simulink model "evse_full_shit"  (R2023b)
settings: Solver=VariableStepAuto  StartTime=0.0  StopTime=5  RelTol=1e-3
settings Model: Creator=dawid  LastModifiedBy=dawid
settings OptimizationCC: BooleanDataType=off

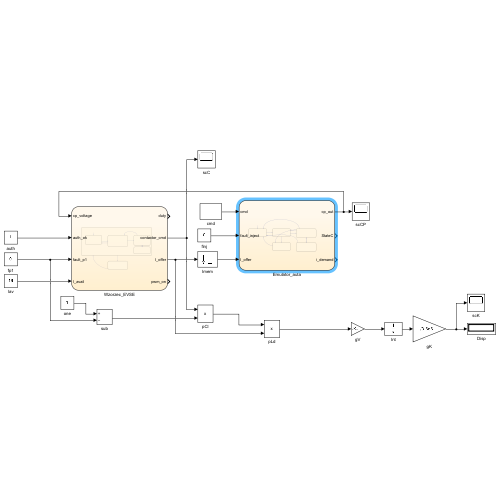
[thumbnail: Simulink's stored preview of the top-level diagram]
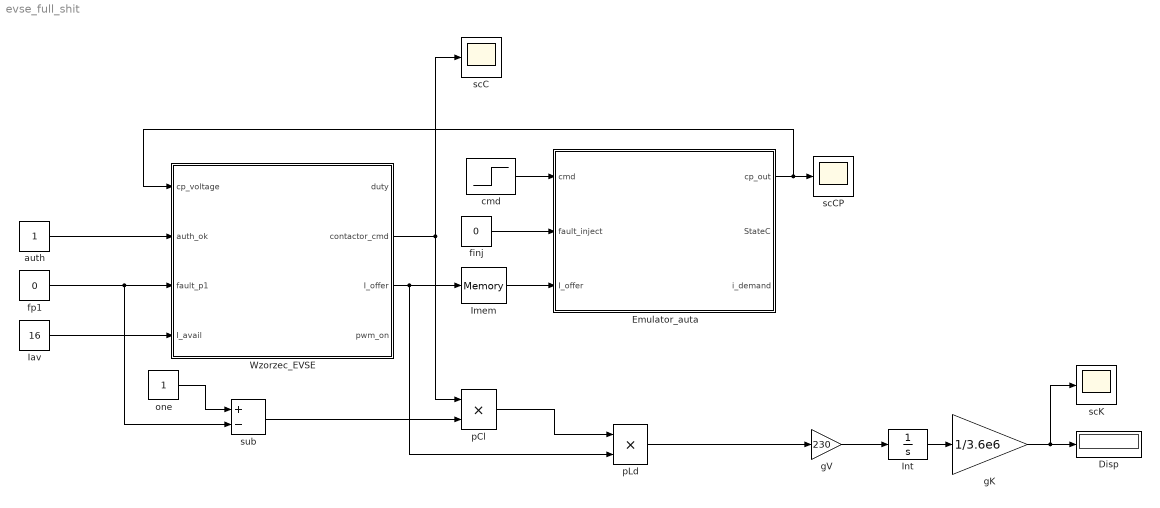
== system evse_full_shit ==
  Disp : Display
  Emulator_auta : Stateflow chart  TreatAsAtomicUnit=on
  Iav : Constant  Value=16
  Imem : Memory
  Int : Integrator
  Wzorzec_EVSE : Stateflow chart  TreatAsAtomicUnit=on
  auth : Constant
  cmd : Step  Time=2  Before=1  After=2  SampleTime=0
  finj : Constant  Value=0
  fp1 : Constant  Value=0
  gK : Gain  Gain=1/3.6e6
  gV : Gain  Gain=230
  one : Constant
  pCl : Product
  pLd : Product
  scC : Scope
  scCP : Scope
  scK : Scope
  sub : Sum  Inputs=+-
  wires:
  one/1 -> sub/1
  finj/1 -> Emulator_auta/2(fault_inject)
  auth/1 -> Wzorzec_EVSE/2(auth_ok)
  cmd/1 -> Emulator_auta/1(cmd)
  Iav/1 -> Wzorzec_EVSE/4(I_avail)
  Wzorzec_EVSE/2(contactor_cmd) -> pCl/1, scC/1
  fp1/1 -> Wzorzec_EVSE/3(fault_p1), sub/2
  Wzorzec_EVSE/3(I_offer) -> Imem/1, pLd/2
  sub/1 -> pCl/2
  Imem/1 -> Emulator_auta/3(I_offer)
  pCl/1 -> pLd/1
  Emulator_auta/1(cp_out) -> Wzorzec_EVSE/1(cp_voltage), scCP/1
  pLd/1 -> gV/1
  gV/1 -> Int/1
  Int/1 -> gK/1
  gK/1 -> Disp/1, scK/1

== stateflow chart evse_full_shit/Wzorzec_EVSE ==
  state Operating
    state Idle
      entry: pwm_on=0; duty=0; contactor_cmd=0; I_offer=0;
    state Detected
      entry: pwm_on=1; I_offer=I_avail; duty=max(10,min(85,I_offer/0.6)); contactor_cmd=0;
    state Charging
      entry: contactor_cmd=1;
      during: I_offer=I_avail; duty=max(10,min(85,I_offer/0.6));
    state Ventilation
      entry: contactor_cmd=1;
    Charging -> Detected [order 1] : [cp_voltage>7.5 && cp_voltage<10.5]
    (default) -> Idle
    Detected -> Charging [order 1] : [cp_voltage>4.5 && cp_voltage<7.5 && auth_ok==1]
    Idle -> Detected : [cp_voltage>7.5 && cp_voltage<10.5 && I_avail>0]
    Detected -> Idle [order 2] : [cp_voltage>10.5]
    Charging -> Ventilation [order 2] : [cp_voltage>1.5 && cp_voltage<4.5]
    Ventilation -> Charging : [cp_voltage>4.5 && cp_voltage<7.5]
  state Tripped
    entry: contactor_cmd=0; pwm_on=0; duty=0;
  Tripped -> Operating : [fault_p1==0 && cp_voltage>1.5]
  Operating -> Tripped : [fault_p1==1 || cp_voltage<1.5]
  data: cp_voltage input; auth_ok input; fault_p1 input; I_avail input; duty output; contactor_cmd output; I_offer output; pwm_on output

== stateflow chart evse_full_shit/Emulator_auta ==
  state A_Unplugged
    entry: cp_out=12; StateC=0; i_demand=0;
  state B_Connected
    entry: cp_out=9; StateC=0; i_demand=0;
  state C_Ready
    entry: cp_out=6; StateC=1; i_demand=min(I_offer,32);
  state Fault
    entry: cp_out=0; StateC=0; i_demand=0;
  state D_Vent
    entry: cp_out=3; StateC=1; i_demand=min(I_offer,32);
  C_Ready -> A_Unplugged [order 3] : [cmd==0]
  (default) -> A_Unplugged
  C_Ready -> B_Connected [order 1] : [cmd==3]
  C_Ready -> Fault [order 4] : [fault_inject==1]
  A_Unplugged -> B_Connected : [cmd==1]
  B_Connected -> C_Ready [order 1] : [cmd==2]
  D_Vent -> A_Unplugged [order 2] : [cmd==0]
  B_Connected -> A_Unplugged [order 2] : [cmd==0]
  Fault -> A_Unplugged : [fault_inject==0]
  B_Connected -> Fault [order 3] : [fault_inject==1]
  C_Ready -> D_Vent [order 2] : [cmd==4]
  D_Vent -> C_Ready [order 1] : [cmd==2]
  data: cmd input; fault_inject input; I_offer input; cp_out output; StateC output; i_demand output
